simulink model "Follower_Agent"  (R2014b)
settings: Solver=ode3  SolverMode=SingleTasking  StartTime=0.0  StopTime=10.0  FixedStep=sampleTimes.main  RelTol=1e-3
model workspace (MAT data in the model file):
  vehicle = 0
undefined symbols (not defined in the file or in its folder): delays, sampleTimes
libraries: simulink x18
(part 2 of 2)

== system Follower_Agent/Data Models/Sensor Model1/Sense each vehicle/Radar Model1/CG to Sensor transform ==
  dPsi : Inport
  distance : Inport  Port=2
  angle : Inport  Port=3
  MATLAB Function : MATLAB Function  TreatAsAtomicUnit=on
  range : Outport
  azimuth : Outport  Port=2
  wires:
  distance/1 -> MATLAB Function/1(d)
  angle/1 -> MATLAB Function/2(theta)
  dPsi/1 -> MATLAB Function/3(dpsi)
  MATLAB Function/1(d_r) -> range/1
  MATLAB Function/2(theta_c) -> azimuth/1

== system Follower_Agent/Data Models/Sensor Model1/Sense each vehicle/Radar Model1/Norm ==
  In1 : Inport
  Math Function : Math  Operator=square  SaturateOnIntegerOverflow=on
  Sqrt : Sqrt  SaturateOnIntegerOverflow=on
  Sum of Elements : Sum  Inputs=+
  Out1 : Outport
  wires:
  Math Function/1 -> Sum of Elements/1
  Sum of Elements/1 -> Sqrt/1
  Sqrt/1 -> Out1/1
  In1/1 -> Math Function/1

== system Follower_Agent/Data Models/Sensor Model1/Sense each vehicle/Radar Model1/Wrap to Pi ==
  In : Inport
  Bias : Bias  Bias=pi
  Bias1 : Bias  Bias=-pi
  Constant : Constant  Value=2*pi
  Math Function : Math  Operator=mod  SaturateOnIntegerOverflow=on
  Out : Outport
  wires:
  In/1 -> Bias/1
  Bias/1 -> Math Function/1
  Math Function/1 -> Bias1/1
  Bias1/1 -> Out/1
  Constant/1 -> Math Function/2

== system Follower_Agent/Data Models/Sensor Model1/Sense each vehicle/Radar Model1/Wrap to Pi1 ==
  In : Inport
  Bias : Bias  Bias=pi
  Bias1 : Bias  Bias=-pi
  Constant : Constant  Value=2*pi
  Math Function : Math  Operator=mod  SaturateOnIntegerOverflow=on
  Out : Outport
  wires:
  In/1 -> Bias/1
  Bias/1 -> Math Function/1
  Math Function/1 -> Bias1/1
  Bias1/1 -> Out/1
  Constant/1 -> Math Function/2

== system Follower_Agent/Data Models/Sensor Model1/Sense each vehicle/Radar Model1/Wrap to Pi2 ==
  In : Inport
  Bias : Bias  Bias=pi
  Bias1 : Bias  Bias=-pi
  Constant : Constant  Value=2*pi
  Math Function : Math  Operator=mod  SaturateOnIntegerOverflow=on
  Out : Outport
  wires:
  Constant/1 -> Math Function/2
  Bias1/1 -> Out/1
  Math Function/1 -> Bias1/1
  Bias/1 -> Math Function/1
  In/1 -> Bias/1

== system Follower_Agent/Follower Vehicle Control/Platoon Steering Control1/Calculate lateral error1/Subsystem1/Wrap to Pi2 ==
  In : Inport
  Bias : Bias  Bias=pi
  Bias1 : Bias  Bias=-pi
  Constant : Constant  Value=2*pi
  Math Function : Math  Operator=mod  SaturateOnIntegerOverflow=on
  Out : Outport
  wires:
  Constant/1 -> Math Function/2
  Bias1/1 -> Out/1
  Math Function/1 -> Bias1/1
  Bias/1 -> Math Function/1
  In/1 -> Bias/1

== matlab function Follower_Agent/Assignment/MATLAB Function ==
  data: dataIn input Bus: VehicleBus size=10; V2Vin input Bus: V2VBus size=10; myV2V input Bus: V2VBus size=1; brake input size=1; throttle input; gear input; clutch input; steering input; dataOut output Bus: VehicleBus size=10; vehicle input; V2Vout output Bus: V2VBus size=10
function [dataOut, V2Vout]  = fcn(dataIn, V2Vin, myV2V, brake,throttle,gear,clutch,steering, vehicle)
%#codegen

dataOut = dataIn;
dataOut(vehicle).control.brake = brake;
dataOut(vehicle).control.throttle = throttle;
dataOut(vehicle).control.clutch = clutch;
dataOut(vehicle).control.steering = steering;
dataOut(vehicle).control.gear = gear;

V2Vout = V2Vin;
V2Vout(vehicle) = myV2V;

== matlab function Follower_Agent/Selectors/MATLAB Function ==
  data: egoTruth output Bus: VehicleBus size=1; leaderV2V output Bus: V2VBus size=1; precedingV2V output Bus: V2VBus size=1; data input Bus: VehicleBus size=10; V2V input Bus: V2VBus size=10; vehicle input
function [egoTruth, leaderV2V, precedingV2V] = fcn(data, V2V, vehicle)
%#codegen

if (vehicle > 1)
    precedingV2V = V2V(vehicle-1);
else
    error('There is no preceeding vehicle!');
end
egoTruth = data(vehicle);

leaderV2V = V2V(1);

== matlab function Follower_Agent/Follower Vehicle Control/Variant Subsystem/Agent Control/MATLAB Function1 ==
  data: buf output; ego_timestamp input double; ego_distance input double; ego_speed input double; ego_acceleration input double; ego_lateralAcceleration input double; ego_yawRate input double; ego_heading input double; ego_range input double; ego_azimuth input double; ego_lateralPosition input double; ego_headingError input double; ego_roadCurvature input double; leader_latency input double; leader_distance input double; leader_speed input double; leader_acceleration input double; leader_lateralAcceleration input double; leader_yawRate input double; leader_heading input double; leader_lateralPosition input double; leader_headingError input double; leader_roadCurvature input double; pre_platoonID input double; pre_latency input double; pre_distance input double; pre_speed input double; pre_acceleration input double; pre_lateralAcceleration input double; pre_yawRate input double; pre_heading input double; pre_range input double; pre_azimuth input double; pre_lateralPosition input double
function buf  = fcn(...
ego_timestamp, ego_distance, ego_speed, ego_acceleration, ...
ego_lateralAcceleration, ego_yawRate, ego_heading, ego_range, ego_azimuth, ...
ego_lateralPosition, ego_headingError, ego_roadCurvature, ...
leader_latency, leader_distance, leader_speed, leader_acceleration, ...
leader_lateralAcceleration, leader_yawRate, leader_heading, ...
leader_lateralPosition, leader_headingError, leader_roadCurvature, ...
pre_platoonID, pre_latency, pre_distance, pre_speed, pre_acceleration, ...
pre_lateralAcceleration, pre_yawRate, pre_heading, pre_range, pre_azimuth, ...
pre_lateralPosition)
%#codegen

buf = zeros(33*8,1,'uint8');

n = 0;

buf(8*n + (1:8)) = typecast(ego_timestamp,'uint8'); n = n + 1;
buf(8*n + (1:8)) = typecast(ego_distance,'uint8'); n = n + 1;
buf(8*n + (1:8)) = typecast(ego_speed,'uint8'); n = n + 1;
buf(8*n + (1:8)) = typecast(ego_acceleration,'uint8'); n = n + 1;
buf(8*n + (1:8)) = typecast(ego_lateralAcceleration,'uint8'); n = n + 1;
buf(8*n + (1:8)) = typecast(ego_yawRate,'uint8'); n = n + 1;
buf(8*n + (1:8)) = typecast(ego_heading,'uint8'); n = n + 1;
buf(8*n + (1:8)) = typecast(ego_range,'uint8'); n = n + 1;
buf(8*n + (1:8)) = typecast(ego_azimuth,'uint8'); n = n + 1;
buf(8*n + (1:8)) = typecast(ego_lateralPosition,'uint8'); n = n + 1;
buf(8*n + (1:8)) = typecast(ego_headingError,'uint8'); n = n + 1;
buf(8*n + (1:8)) = typecast(ego_roadCurvature,'uint8'); n = n + 1;
buf(8*n + (1:8)) = typecast(leader_latency,'uint8'); n = n + 1;
buf(8*n + (1:8)) = typecast(leader_distance,'uint8'); n = n + 1;
buf(8*n + (1:8)) = typecast(leader_speed,'uint8'); n = n + 1;
buf(8*n + (1:8)) = typecast(leader_acceleration,'uint8'); n = n + 1;
buf(8*n + (1:8)) = typecast(leader_lateralAcceleration,'uint8'); n = n + 1;
buf(8*n + (1:8)) = typecast(leader_yawRate,'uint8'); n = n + 1;
buf(8*n + (1:8)) = typecast(leader_heading,'uint8'); n = n + 1;
buf(8*n + (1:8)) = typecast(leader_lateralPosition,'uint8'); n = n + 1;
buf(8*n + (1:8)) = typecast(leader_headingError,'uint8'); n = n + 1;
buf(8*n + (1:8)) = typecast(leader_roadCurvature,'uint8'); n = n + 1;
buf(8*n + (1:8)) = typecast(pre_platoonID,'uint8'); n = n + 1;
buf(8*n + (1:8)) = typecast(pre_latency,'uint8'); n = n + 1;
buf(8*n + (1:8)) = typecast(pre_distance,'uint8'); n = n + 1;
buf(8*n + (1:8)) = typecast(pre_speed,'uint8'); n = n + 1;
buf(8*n + (1:8)) = typecast(pre_acceleration,'uint8'); n = n + 1;
buf(8*n + (1:8)) = typecast(pre_lateralAcceleration,'uint8'); n = n + 1;
buf(8*n + (1:8)) = typecast(pre_yawRate,'uint8'); n = n + 1;
buf(8*n + (1:8)) = typecast(pre_heading,'uint8'); n = n + 1;
buf(8*n + (1:8)) = typecast(pre_range,'uint8'); n = n + 1;
buf(8*n + (1:8)) = typecast(pre_azimuth,'uint8'); n = n + 1;
buf(8*n + (1:8)) = typecast(pre_lateralPosition,'uint8');

== matlab function Follower_Agent/Data Models/Sensor Model1/MATLAB Function ==
  data: ego input; distances output size=10; cars input; angles output size=10
function [distances,angles] = RadarSensor(ego,cars)
%#codegen

% Some data
CarLength = 5;
CarWidth = 2;
maxAzimuth = pi/3;
maxDistance = 100;

% Assume cars are homogenous and sensor is on front bumper
% Calculate sensor position in global coordinates
h_ego = ego.data.angle(3);
P_ego = ego.data.position(1:2) ...
    + [cos(h_ego) -sin(h_ego); sin(h_ego) cos(h_ego)] * [CarLength/2; 0];

% Initialise variables for distance and angle data
% Angle matrix includes three values per car:
%   1: Minimum detectable extremity
%   2: Angle to centre of rear bumper 
%   3: Maximum detectable extremity
allDistances = zeros(length(cars),1);
allAngles = zeros(length(cars),3);

% Loop over all vehicles and calculate sensor readings assuming no
% occlusion problems (i.e. sensor can see through other cars)
for i=1:length(cars)
    % Ignore non-simulated vehicles and self
    if cars(i).data.position(1) == 0 ...
            || (cars(i).data.position(1) == ego.data.position(1) ...
            && cars(i).data.position(2) == ego.data.position(2))
        continue;
    end
    
    % Compute the corner points of the vehicle in global coordinates
    corners = [ CarLength/2 -CarLength/2 -CarLength/2 CarLength/2
                CarWidth/2 CarWidth/2 -CarWidth/2 -CarWidth/2 ];
    h = cars(i).data.angle(3);
    P = repmat(cars(i).data.position(1:2), [1 4]) ...
        + [cos(h) -sin(h); sin(h) cos(h)] * corners;
    
    % Calculate the relative position of the corner points to the ego
    % sensor
    dP = P - repmat(P_ego,[1 4]);
    
    % Calculate the (relative) angles to each corner point and extremities
    theta = atan2(dP(2,:),dP(1,:)) - h_ego;
    theta = mod(theta + pi,2*pi) - pi;
    minT = min(theta);
    maxT = max(theta);
    
    % Calculate the relative position of the centre of the rear bumper
    dP_rb = mean(dP(:,2:3),2);
   
    % Calculate the distance to the rear bumper
    d_rb = sqrt(dP_rb(1)^2 + dP_rb(2)^2);
    
    % Check whether we are within sensor limits
    if abs(minT) < maxAzimuth && abs(maxT) < maxAzimuth && d_rb < maxDistance
        allAngles(i,:) = [ minT ...
            mod((atan2(dP_rb(2),dP_rb(1)) - h_ego)+pi,2*pi)-pi ...
            maxT ];
        allDistances(i) = d_rb;
    end
    
end

% Now account for occluded vehicles. Assume sensor has to see both extremes
% of a vehicle in order to measure it

% Firstly, filter out zeros
nonZeroIdx = allDistances > 0;
nonZeroDistances = allDistances(nonZeroIdx);
nonZeroAngles = allAngles(nonZeroIdx,:);

% Initialise a boolean array which will be used to select those vehicles
% which are visible
visibleIdx = logical(ones(length(nonZeroDistances),1));

% Loop over all vehicles
for i=1:length(nonZeroDistances)
    % Loop over all other vehicles
    for j=1:length(nonZeroDistances)
        if i == j
            continue;
        end
        
        % If a vehicle is further than another, and either of its angular
        % extemities is within the other vehicles, then we say it is
        % occluded and not visible to the ego vehicle
        if nonZeroDistances(i) > nonZeroDistances(j) ...
                && ((nonZeroAngles(i,1) > nonZeroAngles(j,1) ...
                && nonZeroAngles(i,1) < nonZeroAngles(j,3)) ...
                || (nonZeroAngles(i,3) > nonZeroAngles(j,1) ...
                && nonZeroAngles(i,3) < nonZeroAngles(j,3)))
            visibleIdx(i) = false;
            break;
        end
    end
end

% Output non-ocluded measurements of distance and angle to rear-bumper
distances = nonZeroDistances(visibleIdx);
angles = nonZeroAngles(visibleIdx,2);

== matlab function Follower_Agent/Data Models/Sensor Model1/Occlusion ==
  data: distances input size=10; measOut output; angles input size=10; measIn input
function measOut = EgoMeasurmentOccluded(distances, angles, measIn)
%#codegen

measOut = measIn;
if ~isempty(angles)
    deviationFromCentre = abs(angles);

    [deviation, i] = min(deviationFromCentre);

    if distances(i) < 15 && deviation < pi/18
        measOut = measIn * 0;
    end
end

== matlab function Follower_Agent/Follower Vehicle Control/Platoon Steering Control1/Curvature ==
  data: w input; V input; c output
function c = calcCurvature(w, V)
%#codegen

if V < 1
    V = 1;
end

c = w/V;

== matlab function Follower_Agent/Follower Vehicle Control/Platoon Steering Control1/Delay Leader/MATLAB Function1 ==
  data: l input; y output; e input; s input
function y = fcn(l,e,s)
%#codegen

n = 1000;
persistent S D;

if isempty(S)
    S = ones(n,1)*s;
    D = linspace(0.98*l,0.99*l,n);
end

D(1:(end-1)) = D(2:end);
D(end) = l;

S(1:(end-1)) = S(2:end);
S(end) = s;

[t i] = min(abs(D-e));

y = S(i);

== matlab function Follower_Agent/Data Models/Sensor Model1/Sense each vehicle/Radar Model1/CG to Sensor transform/MATLAB Function ==
  data: d input; d_r output; theta input; dpsi input; theta_c output
function [d_r, theta_c] = fcn(d,theta,dpsi)
%#codegen

lb = 2.5;
lr = 2.5;
lc = 2.5;


A = d*sin(theta)/sin(dpsi);
B = d*sin(dpsi-theta)/sin(dpsi);

if (A-lb)^2 + (B-lr)^2 + 2*(A-lb)*(B-lr)*cos(dpsi) > 0
    d_r = sqrt((A-lb)^2 + (B-lr)^2 + 2*(A-lb)*(B-lr)*cos(dpsi));
else
    d_r = sqrt(d^2 + (lb+lr)^2 - 2*d*(lb+lr)*cos(theta));
end

if (A-lb)^2 + (B-lc)^2 + 2*(A-lb)*(B-lc)*cos(dpsi) > 0
    d_c = sqrt((A-lb)^2 + (B-lc)^2 + 2*(A-lb)*(B-lc)*cos(dpsi));
else
    d_c = sqrt(d^2 + (lb+lc)^2 - 2*d*(lb+lc)*cos(theta));
end

if d_c == 0
    theta_c = 0;
else
    theta_c = asin(sin(dpsi)*(A-lb)/d_c);
end

== matlab function Follower_Agent/Data Models/Sensor Model1/Closest ==
  data: All input Bus: SensorData size=10; Closest output Bus: SensorData; v input; i output
function [Closest, i] = fcn(All, v)
%#codegen

minR = Inf;
j = 1;

for i=1:length(All)
    if (i ~= v && All(i).range > 0 && All(i).range < minR)
        minR = All(i).range;
        j = i;
    end
end

%if (j == 0)
%    error('No valid radar data found!');
%end

Closest = All(j);
i = j;

== matlab function Follower_Agent/Follower Vehicle Control/Platoon Speed Control/MATLAB Function ==
  data: C1 input; d input; w input; xdd_p input; v_l input; xdd_c output; xdd_l input; eps input; epsd input; v input
function xdd_c = fcn(C1, d, w, xdd_p, v_l, xdd_l, eps, epsd, v)
%#codegen

% From Rajamani - Vehicle Dynamics and Control

xdd_c = (1-C1)*xdd_p + C1*xdd_l - (2*d - C1*(d + sqrt(d*d - 1)))*w*epsd ...
    - (d + sqrt(d*d - 1))*w*C1*(v-v_l) - w*w*eps;

== matlab function Follower_Agent/Follower Vehicle Control/Platoon Steering Control1/Delay Leader/MATLAB Function2 ==
  data: l input; y output; e input; s input
function y = fcn(l,e,s)
%#codegen

n = 1000;
persistent S D;

if isempty(S)
    S = ones(n,1)*s;
    D = linspace(0.98*l,0.99*l,n);
end

D(1:(end-1)) = D(2:end);
D(end) = l;

S(1:(end-1)) = S(2:end);
S(end) = s;

[t i] = min(abs(D-e));

y = S(i);

== matlab function Follower_Agent/Data Models/Sensor Model1/Sense each vehicle/Radar Model1/MATLAB Function ==
  data: ego input; distance output; car input; angle output
function [distance,angle] = RadarSensor(ego,car)
%#codegen

% Some data
CarLength = 5;
CarWidth = 2;
maxAzimuth = pi/3;
maxDistance = 100;

% Assume cars are homogenous and sensor is on front bumper
% Calculate sensor position in global coordinates
h_ego = ego.data.angle(3);
P_ego = ego.data.position(1:2) ...
    + [cos(h_ego) -sin(h_ego); sin(h_ego) cos(h_ego)] * [CarLength/2; 0];

% Loop over all vehicles and calculate sensor readings assuming no
% occlusion problems (i.e. sensor can see through other cars)
    
    % Compute the corner points of the vehicle in global coordinates
    corners = [ CarLength/2 -CarLength/2 -CarLength/2 CarLength/2
                CarWidth/2 CarWidth/2 -CarWidth/2 -CarWidth/2 ];
    h = car.data.angle(3);
    P = repmat(car.data.position(1:2), [1 4]) ...
        + [cos(h) -sin(h); sin(h) cos(h)] * corners;
    
    % Calculate the relative position of the corner points to the ego
    % sensor
    dP = P - repmat(P_ego,[1 4]);
    
    % Calculate the (relative) angles to each corner point and extremities
    theta = atan2(dP(2,:),dP(1,:)) - h_ego;
    minT = min(theta);
    maxT = max(theta);
    
    % Calculate the relative position of the centre of the rear bumper
    %dP_rb = mean(dP(:,2:3),2);
    dP_rb = car.data.position(1:2) + [cos(h) -sin(h); sin(h) cos(h)] * [-CarLength/2; 0] - P_ego;
   
    % Calculate the distance to the rear bumper
    d_rb = sqrt(dP_rb(1)^2 + dP_rb(2)^2);
    
    angle = (atan2(dP_rb(2),dP_rb(1)) - h_ego);
    distance = d_rb;
end

== matlab function Follower_Agent/Follower Vehicle Control/Platoon Steering Control1/Delay Leader/MATLAB Function3 ==
  data: l input; y output; e input; s input
function y = fcn(l,e,s)
%#codegen

n = 1000;
persistent S D;

if isempty(S)
    S = ones(n,1)*s;
    D = linspace(0.98*l,0.99*l,n);
end

D(1:(end-1)) = D(2:end);
D(end) = l;

S(1:(end-1)) = S(2:end);
S(end) = s;

[t i] = min(abs(D-e));

y = S(i);

== matlab function Follower_Agent/Follower Vehicle Control/Platoon Steering Control1/Calculate lateral error1/Subsystem1/MATLAB Function ==
  data: d output; d_r input; theta_c input; theta output; dpsi input
function [d, theta] = fcn(d_r,theta_c,dpsi)
%#codegen

% Calculate distance and angle between centre of masses of two vehicles,
% assuming that theta_c is the angle measured from a camera (located lc
% distance ahead of the centre of mass of the follower vehicle) to the
% centre of the rear bumper of the preceding vehicle (a distance lb behind
% the centre of mass of the preceding vehicle, and that d is the distance
% measured from a radar sensor (located a distance lr ahead of the centre
% of mass of the following vehicle), to the same point on the bumper

lb = 2.5;   % Distance of rear bumper from CoM of preceding vehicle (estimated)
lr = 2.5;   % Distance of radar (distance sensor) from CoM of following vehicle (estimated)
lc = 2.5;     % Distance of camera (angle sensor) from CoM of following vehicle (estimated)

d_c = (lr -lc)*cos(theta_c) + sqrt(d_r^2 - (lr-lc)^2*sin(theta_c)^2);
theta_b = atan(d_c*sin(theta_c)/(d_c*cos(theta_c) + lc));

d_b = sqrt(d_c^2 + lc^2 + 2*d_c*lc*cos(theta_b));

d = sqrt(d_b^2 + lb^2 + 2*d_b*lb*cos(dpsi-theta_b));
theta = dpsi - atan((d_b*sin(dpsi-theta_b))/(d_b*cos(dpsi-theta_b)+lb));

== matlab function Follower_Agent/Follower Vehicle Control/Platoon Steering Control1/MATLAB Function ==
  data: a input; b input; c input; lambda input; V input; ydd_c output; ydd_p input; ydd_l input; eps input; epsd input; dy_l input; dv_l input
function ydd_c = fcn(a, b, c, lambda, V, ydd_p, ydd_l, eps, epsd,dy_l, dv_l)
%#codegen

if V < 1
    V = 1;
end

ydd_c = 1/(1+b)*(ydd_p + b*ydd_l - (a + lambda)*epsd/V^2 - a*lambda*eps/V^2 - (lambda*b+c)*dv_l/V^2 - lambda*c*dy_l/V^2);

== matlab function Follower_Agent/Data Models/Sensor Model1/Target ==
  data: distances input size=10; distance output; angles input size=10; angle output
function [distance, angle] = TargetOfInterest(distances, angles)
%#codegen

if isempty(angles)
    distance = 100;
    angle = 0;
else
    deviationFromCentre = abs(angles);

    [~, i] = min(deviationFromCentre);

    angle = angles(i);
    distance = distances(i);
end

== matlab function Follower_Agent/Follower Vehicle Control/Variant Subsystem/Agent Control/Message Parser/MATLAB Function ==
  data: buf input uint8 size=[16 1]; speed_control output; steering_control output; spacing output
function [speed_control, steering_control, spacing] = fcn(buf)
%#codegen

persistent speed_control_last steering_control_last spacing_last;

if (isempty(speed_control_last))
    speed_control_last = false;
    steering_control_last = false;
    spacing_last = 6;
end

command_number = int32(0);
num_args = int32(0);
arg = 0;

command_number = typecast(buf(1:4),'int32');
num_args = typecast(buf(5:8), 'int32');

switch (command_number)
    case 1  % speed_controller
        if (num_args ~= 1)
            error('Not enough arguments for speed_controller message');
        end
        arg = typecast(buf(9:16),'double');
        speed_control_last = logical(arg);
    case 2 % steering_controller
        if (num_args ~= 1)
            error('Not enough arguments for steering_controller message');
        end
        arg = typecast(buf(9:16),'double');
        steering_control_last = logical(arg);
    case 3 % set_spacing
        if (num_args ~= 1)
            error('Not enough arguments for set_spacing message');
        end
        arg = typecast(buf(9:16),'double');
        spacing_last = arg;
end

speed_control = speed_control_last;
steering_control = steering_control_last;
spacing = spacing_last;

== stateflow chart Follower_Agent/Follower Vehicle Control/Variant Subsystem/Non-Agent Control/Enable Platooning ==
  state NotPlatooning
    en: speedControl = logical(0); steeringControl = logical(0); lane = int32(0); spacing = 6;
    state GainSpeed
    state CloseDistance
      en: speedControl = logical(1);
    (default) -> GainSpeed
    GainSpeed -> CloseDistance : after(10,sec)[prePlatooning>0 ...
        |  && speed>10]
  state Platooning
    en: steeringControl = logical(1);
  state PreLeave1
    en: spacing = 20;
  state PreLeave2
    en: lane = int32(2);
  state Leave
    en: steeringControl = logical(0); speedControl = logical(0);
  (default) -> NotPlatooning
  CloseDistance -> Platooning : [distance < 20]
  Platooning -> PreLeave1 : after(30000,sec)
  PreLeave1 -> PreLeave2 : [distance > 15]
  PreLeave2 -> Leave : after(30,sec)[abs(azimuth)>pi/36]
  data: speedControl output boolean; speed input; distance input; azimuth input; prePlatooning input int32; steeringControl output boolean; lane output; spacing output
